simulink model "FC_int_RT"  (R2025b)
settings: Solver=FixedStepAuto  StartTime=0.0  StopTime=350  FixedStep=.1  RelTol=1e-3
values from neighbouring files (symbols this model uses):
  e_max = 0.9    [Fuzzy_control.m]
  ed_max = 0.36    [Fuzzy_control.m]
  ref_min = -3    [Fuzzy_control.m]
  t1 = 10    [Fuzzy_control.m]
  t2 = 150    [Fuzzy_control.m]
libraries: fuzblock x1
settings Model: Creator=Uros  LastModifiedBy=Uros

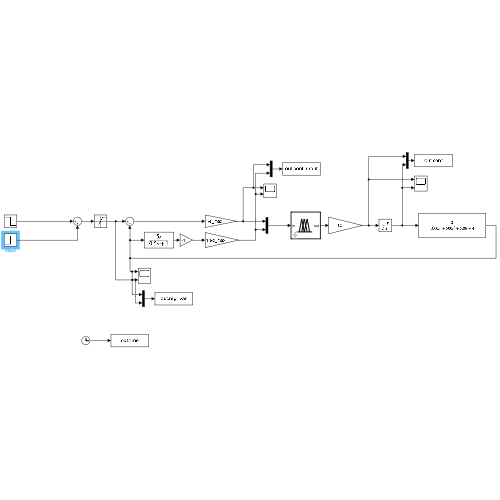
[thumbnail: Simulink's stored preview of the top-level diagram]
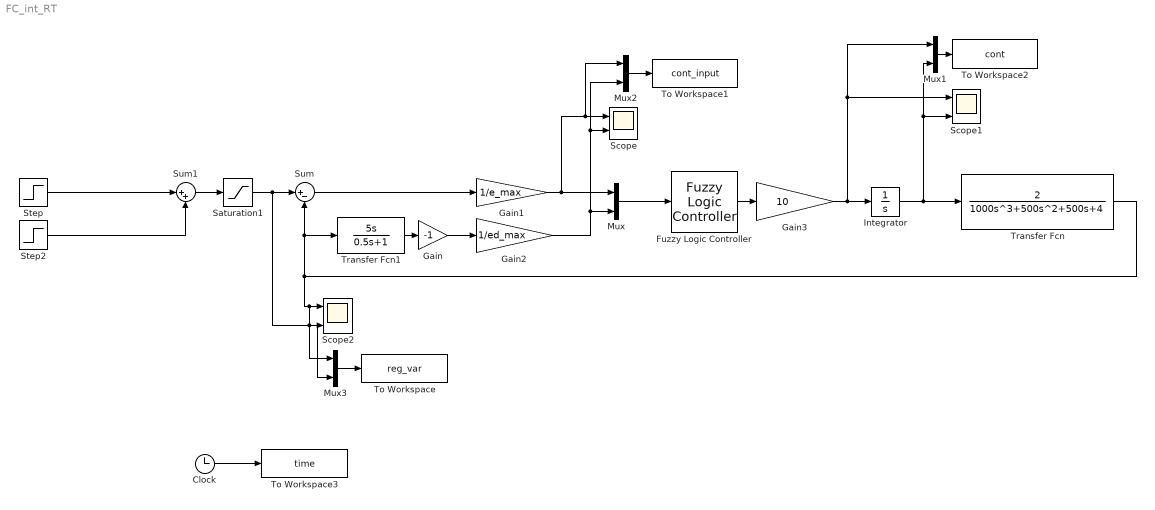
== system FC_int_RT ==
  Clock : Clock
  Fuzzy Logic Controller : fuzblock/Fuzzy Logic  Controller  FIS=FIS_RT  OutputSampleNumber=101  DataType=double  UseLookupTable=off  NumBreakpoints=10  FuzzifiedInputs=off  RuleFiringStrengths=off  RuleOutputs=off  AggregatedOutputs=off  SimulateUsing=Interpreted execution  OutOfRangeInputValueMessage=warning  NoRuleFiredMessage=warning  EmptyOutputFuzzySetMessage=warning
  Gain : Gain  Gain=-1
  Gain1 : Gain  Gain=1/e_max
  Gain2 : Gain  Gain=1/ed_max
  Gain3 : Gain  Gain=10
  Integrator : Integrator  LimitOutput=on  UpperSaturationLimit=15  LowerSaturationLimit=-15
  Mux{,1..3} (4 alike) : Mux  Inputs=2
  Saturation1 : Saturate  UpperLimit=3  LowerLimit=-3
  Scope : Scope  NumInputPorts=2
      settings: ActiveDisplayYMinimum=-1.1348290996811747  ActiveDisplayYMaximum=1.0223275456603849
  Scope1 : Scope  NumInputPorts=2
      settings: ActiveDisplayYMinimum=-18.75  ActiveDisplayYMaximum=18.75
  Scope2 : Scope  NumInputPorts=2
      settings: ActiveDisplayYMinimum=-3.75  ActiveDisplayYMaximum=3.75  DataLoggingVariableName=ScopeData2
  Step : Step  Time=t1  After=ref_min  SampleTime=0
  Step2 : Step  Time=t2  After=ref_max-ref_min  SampleTime=0
  Sum : Sum  Inputs=|+-
  Sum1 : Sum  Inputs=|++
  To Workspace : ToWorkspace  VariableName=reg_var  SampleTime=-1
      settings: Save2DSignal=2-D array (concatenate along first dimension)
  To Workspace1 : ToWorkspace  VariableName=cont_input  SampleTime=-1
      settings: Save2DSignal=2-D array (concatenate along first dimension)
  To Workspace2 : ToWorkspace  VariableName=cont  SampleTime=-1
      settings: Save2DSignal=2-D array (concatenate along first dimension)
  To Workspace3 : ToWorkspace  VariableName=time  SampleTime=-1
      settings: Save2DSignal=2-D array (concatenate along first dimension)
  Transfer Fcn : TransferFcn  Numerator=[2]  Denominator=[1000 500 500 4]
  Transfer Fcn1 : TransferFcn  Numerator=[5 0]  Denominator=[0.5 1]
  wires:
  Transfer Fcn1/1 -> Gain/1
  Sum/1 -> Gain1/1
  Saturation1/1 -> Mux3/2, Scope2/2, Sum/1
  Gain1/1 -> Mux2/1, Scope/1, Mux/1
  Gain/1 -> Gain2/1
  Gain2/1 -> Mux2/2, Scope/2, Mux/2
  Transfer Fcn/1 -> Mux3/1, Scope2/1, Transfer Fcn1/1, Sum/2
  Gain3/1 -> Mux1/1, Scope1/1, Integrator/1
  Fuzzy Logic Controller/1 -> Gain3/1
  Integrator/1 -> Mux1/2, Scope1/2, Transfer Fcn/1
  Mux/1 -> Fuzzy Logic Controller/1
  Sum1/1 -> Saturation1/1
  Step/1 -> Sum1/1
  Step2/1 -> Sum1/2
  Mux1/1 -> To Workspace2/1
  Mux2/1 -> To Workspace1/1
  Mux3/1 -> To Workspace/1
  Clock/1 -> To Workspace3/1
